simulink model "nonlineardtm"  (R2018b)
settings: configuration reference "Physics" (kept outside this file)
model workspace (MAT data in the model file):
  x0_initialstates = Simulink.Parameter
  x0_initialstates.Value = [0 0 0 0 0 0]
  x0_initialstates.DataType = 'auto'
  x0_initialstates.Dimensions = [1 6]
undefined symbols (not defined in the file): INIT__initialvalues__Vehicle_InitialPitchAngle, INIT__initialvalues__Vehicle_InitialPitchRate_radps, INIT__initialvalues__Vehicle_InitialVelocity_mps__2, INIT__initialvalues__Vehicle_InitialVelocity_mps__3, INIT__initialvalues__Vehicle_InitialYawAngle, INIT__initialvalues__Vehicle_InitialYawRate_radps, tireFL__INERTIAL__m_Wheel_kg, tireFL__SCALING__LCX, tireFL__SCALING__LCY, tireFL__SCALING__LCZ, tireFL__SCALING__LEX, tireFL__SCALING__LEY, tireFL__SCALING__LFZO, tireFL__SCALING__LGAY, tireFL__SCALING__LGAZ, tireFL__SCALING__LHX, tireFL__SCALING__LHY, tireFL__SCALING__LKX, tireFL__SCALING__LKY, tireFL__SCALING__LMPHI, tireFL__SCALING__LMUV, tireFL__SCALING__LMX, tireFL__SCALING__LMY, tireFL__SCALING__LRES, tireFL__SCALING__LS, tireFL__SCALING__LTR, tireFL__SCALING__LVMX, tireFL__SCALING__LVX, tireFL__SCALING__LVY, tireFL__SCALING__LVYKA, tireFL__SCALING__LXAL, tireFL__SCALING__LYKA, tireFR__INERTIAL__m_Wheel_kg, tireFR__SCALING__LCX, tireFR__SCALING__LCY, tireFR__SCALING__LCZ, tireFR__SCALING__LEX, tireFR__SCALING__LEY, tireFR__SCALING__LFZO, tireFR__SCALING__LGAY, tireFR__SCALING__LGAZ, tireFR__SCALING__LHX, tireFR__SCALING__LHY, tireFR__SCALING__LKX, tireFR__SCALING__LKY, tireFR__SCALING__LMPHI, tireFR__SCALING__LMUV, tireFR__SCALING__LMX, tireFR__SCALING__LMY, tireFR__SCALING__LRES, tireFR__SCALING__LS, tireFR__SCALING__LTR, tireFR__SCALING__LVMX, tireFR__SCALING__LVX, tireFR__SCALING__LVY, tireFR__SCALING__LVYKA, tireFR__SCALING__LXAL, tireFR__SCALING__LYKA, tireRL__INERTIAL__m_Wheel_kg, tireRL__SCALING__LCX ... (+71)
libraries: vehdynlibtire_TUM x4, vehdynlibsuspension x2, vrlib x1, vehdynlibeom_TUM x1
(part 1 of 5)
settings Model: DataDictionary=vehicleparameters_vehdynsim.sldd  ParameterArgumentNames=x0_initialstates  OrderedModelArguments=off  Creator=wischnewski  LastModifiedBy=Michael

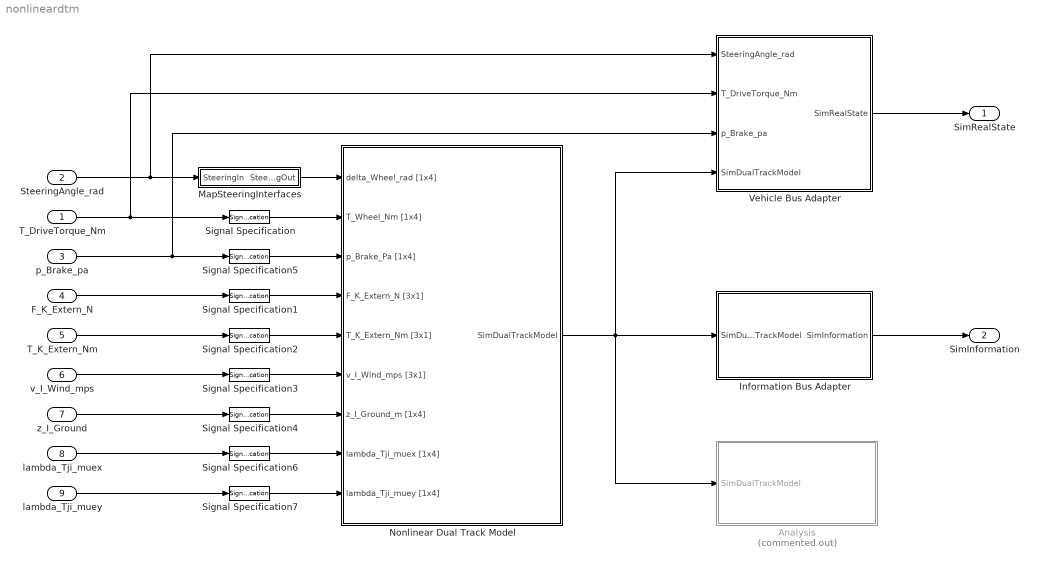
== system nonlineardtm ==
  T_DriveTorque_Nm : Inport  OutDataTypeStr=double
  SteeringAngle_rad : Inport  Port=2  OutDataTypeStr=double
  p_Brake_pa : Inport  Port=3  OutDataTypeStr=double
  F_K_Extern_N : Inport  Port=4  OutDataTypeStr=double
  T_K_Extern_Nm : Inport  Port=5  OutDataTypeStr=double
  v_I_Wind_mps : Inport  Port=6  OutDataTypeStr=double
  z_I_Ground : Inport  Port=7  OutDataTypeStr=double
  lambda_Tji_muex : Inport  Port=8  OutDataTypeStr=double
  lambda_Tji_muey : Inport  Port=9  OutDataTypeStr=double
  Analysis : Subsystem  Commented=on
  Information Bus Adapter : Subsystem
  MapSteeringInterfaces : Subsystem
  Nonlinear Dual Track Model : Subsystem
  Signal Specification{,4..7} (5 alike) : SignalSpecification  Dimensions=[1,4]
  Signal Specification1 : SignalSpecification  Dimensions=[3,1]
  Signal Specification2 : SignalSpecification  Dimensions=[3,1]
  Signal Specification3 : SignalSpecification  Dimensions=[3,1]
  Vehicle Bus Adapter : Subsystem
  SimRealState : Outport  OutDataTypeStr=Bus: SimRealState
  SimInformation : Outport  Port=2  OutDataTypeStr=Bus: SimInformation
  wires:
  Vehicle Bus Adapter/1(SimRealState) -> SimRealState/1
  Nonlinear Dual Track Model/1(SimDualTrackModel) -> Vehicle Bus Adapter/4(SimDualTrackModel), Information Bus Adapter/1(SimDualTrackModel), Analysis/1(SimDualTrackModel)
  Information Bus Adapter/1(SimInformation) -> SimInformation/1
  F_K_Extern_N/1 -> Signal Specification1/1
  T_K_Extern_Nm/1 -> Signal Specification2/1
  v_I_Wind_mps/1 -> Signal Specification3/1
  z_I_Ground/1 -> Signal Specification4/1
  lambda_Tji_muex/1 -> Signal Specification6/1
  lambda_Tji_muey/1 -> Signal Specification7/1
  p_Brake_pa/1 -> Signal Specification5/1, Vehicle Bus Adapter/3("p_Brake_pa ")
  T_DriveTorque_Nm/1 -> Vehicle Bus Adapter/2(T_DriveTorque_Nm), Signal Specification/1
  MapSteeringInterfaces/1(SteeringOut) -> Nonlinear Dual Track Model/1(delta_Wheel_rad [1x4])
  SteeringAngle_rad/1 -> Vehicle Bus Adapter/1(SteeringAngle_rad), MapSteeringInterfaces/1(SteeringIn)
  Signal Specification/1 -> Nonlinear Dual Track Model/2(T_Wheel_Nm [1x4])
  Signal Specification1/1 -> Nonlinear Dual Track Model/4(F_K_Extern_N [3x1])
  Signal Specification2/1 -> Nonlinear Dual Track Model/5(T_K_Extern_Nm [3x1])
  Signal Specification3/1 -> Nonlinear Dual Track Model/6(v_I_Wind_mps [3x1])
  Signal Specification4/1 -> Nonlinear Dual Track Model/7(z_I_Ground_m [1x4])
  Signal Specification5/1 -> Nonlinear Dual Track Model/3(p_Brake_Pa [1x4])
  Signal Specification6/1 -> Nonlinear Dual Track Model/8(lambda_Tji_muex [1x4])
  Signal Specification7/1 -> Nonlinear Dual Track Model/9(lambda_Tji_muey [1x4])

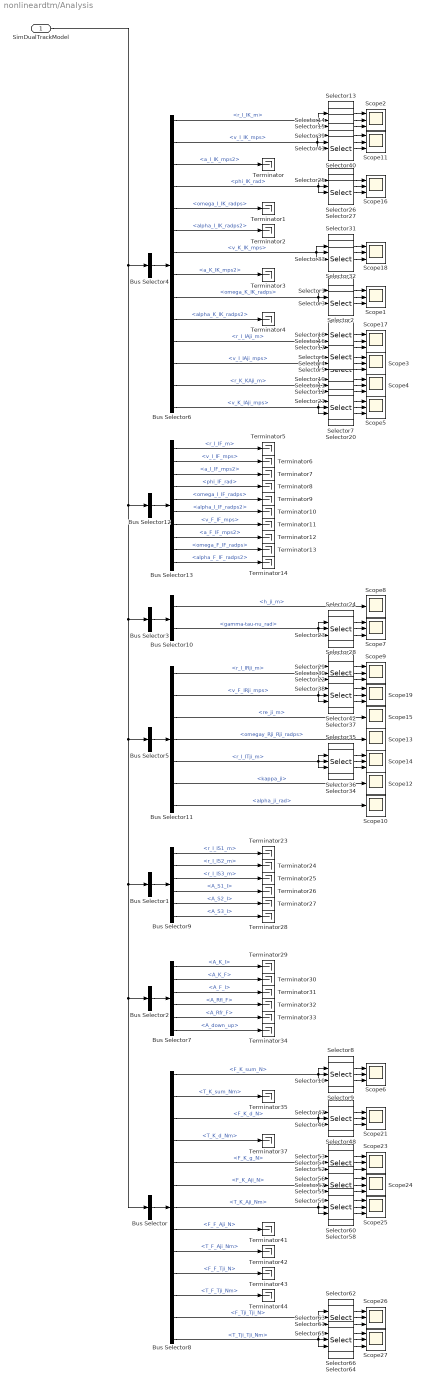
== system nonlineardtm/Analysis ==
  SimDualTrackModel : Inport
  Bus Selector : BusSelector  OutputSignals=SimForce  OutputAsBus=on
  Bus Selector1 : BusSelector  OutputSignals=SimSensor  OutputAsBus=on
  Bus Selector10 : BusSelector  OutputSignals=h_ji_m,gamma-tau-nu_rad
  Bus Selector11 : BusSelector  OutputSignals=r_I_IRji_m,v_F_IRji_mps,re_ji_m,omegay_Rji_Rji_radps,r_I_ITji_m,kappa_ji,alpha_ji_rad
  Bus Selector12 : BusSelector  OutputSignals=SimChassis  OutputAsBus=on
  Bus Selector13 : BusSelector  OutputSignals=r_I_IF_m,v_I_IF_mps,a_I_IF_mps2,phi_IF_rad,omega_I_IF_radps,alpha_I_IF_radps2,v_F_IF_mps,a_F_IF_mps2,omega_F_IF_radps,alpha_F_IF_radps2
  Bus Selector2 : BusSelector  OutputSignals=signal6  OutputAsBus=on
  Bus Selector3 : BusSelector  OutputSignals=SimSuspension  OutputAsBus=on
  Bus Selector4 : BusSelector  OutputSignals=signal1  OutputAsBus=on
  Bus Selector5 : BusSelector  OutputSignals=SimWheel  OutputAsBus=on
  Bus Selector6 : BusSelector  OutputSignals=r_I_IK_m,v_I_IK_mps,a_I_IK_mps2,phi_IK_rad,omega_I_IK_radps,alpha_I_IK_radps2,v_K_IK_mps,a_K_IK_mps2,omega_K_IK_radps,alpha_K_IK_radps2,r_I_IAji_m,v_I_IAji_mps,r_K_KAji_m,v_K_IAji_mps
  Bus Selector7 : BusSelector  OutputSignals=A_K_I,A_K_F,A_F_I,A_Rfl_F,A_Rfr_F,A_down_up
  Bus Selector8 : BusSelector  OutputSignals=F_K_sum_N,T_K_sum_Nm,F_K_d_N,T_K_d_Nm,F_K_g_N,F_K_Aji_N,T_K_Aji_Nm,F_F_Aji_N,T_F_Aji_Nm,F_F_Tji_N,T_F_Tji_Nm,F_Tji_Tji_N,T_Tji_Tji_Nm
  Bus Selector9 : BusSelector  OutputSignals=r_I_IS1_m,r_I_IS2_m,r_I_IS3_m,A_S1_I,A_S2_I,A_S3_I
  Scope{1..7,9,11,14,16..19,21,23..27} (20 alike) : Scope  NumInputPorts=3
  Scope{8,10,12..13,15} (5 alike) : Scope
  Selector{1,8,13,25,31,39,47,53} (8 alike) : Selector  InputPortWidth=3  IndexOptions=Index vector (dialog)  Indices=[1]  OutputSizes=1
  Selector{3,10,15,27,33,41,46,52} (8 alike) : Selector  InputPortWidth=3  IndexOptions=Index vector (dialog)  Indices=[3]  OutputSizes=1
  Selector{4,7,11,16,28,30,36,42,57,60,63,66} (12 alike) : Selector  NumberOfDimensions=2  InputPortWidth=3  IndexOptions=Index vector (dialog),Select all  Indices=2,1  OutputSizes=1,1
  Selector{5,12,17,20,22..23,34,37,55,58,61,64} (12 alike) : Selector  NumberOfDimensions=2  InputPortWidth=3  IndexOptions=Index vector (dialog),Select all  Indices=3,1  OutputSizes=1,1
  Selector{2,9,14,26,32,40,48,54} (8 alike) : Selector  InputPortWidth=3  IndexOptions=Index vector (dialog)  Indices=[2]  OutputSizes=1
  Selector{6,18..19,21,24,29,35,38,56,59,62,65} (12 alike) : Selector  NumberOfDimensions=2  InputPortWidth=3  IndexOptions=Index vector (dialog),Select all  Indices=1,1  OutputSizes=1,1
  Terminator{,1..14,23..35,37,41..44} (33 alike) : Terminator
  wires:
  SimDualTrackModel/1 -> Bus Selector12/1, Bus Selector5/1, Bus Selector/1, Bus Selector2/1, Bus Selector1/1, Bus Selector3/1, Bus Selector4/1
  Bus Selector12/1 -> Bus Selector13/1
  Bus Selector13/1 -> Terminator5/1  "<r_I_IF_m>"
  Bus Selector13/2 -> Terminator6/1  "<v_I_IF_mps>"
  Bus Selector13/3 -> Terminator7/1  "<a_I_IF_mps2>"
  Bus Selector13/4 -> Terminator8/1  "<phi_IF_rad>"
  Bus Selector13/5 -> Terminator9/1  "<omega_I_IF_radps>"
  Bus Selector13/6 -> Terminator10/1  "<alpha_I_IF_radps2>"
  Bus Selector13/7 -> Terminator11/1  "<v_F_IF_mps>"
  Bus Selector13/8 -> Terminator12/1  "<a_F_IF_mps2>"
  Bus Selector13/9 -> Terminator13/1  "<omega_F_IF_radps>"
  Bus Selector13/10 -> Terminator14/1  "<alpha_F_IF_radps2>"
  Bus Selector11/6 -> Scope12/1  "<kappa_ji>"
  Bus Selector11/7 -> Scope10/1  "<alpha_ji_rad>"
  Bus Selector11/4 -> Scope13/1  "<omegay_Rji_Rji_radps>"
  Bus Selector11/3 -> Scope15/1  "<re_ji_m>"
  Bus Selector11/1 -> Selector29/1, Selector30/1, Selector22/1  "<r_I_IRji_m>"
  Bus Selector5/1 -> Bus Selector11/1
  Bus Selector10/1 -> Scope8/1  "<h_ji_m>"
  Bus Selector3/1 -> Bus Selector10/1
  Bus Selector6/11 -> Selector16/1, Selector17/1, Selector18/1  "<r_I_IAji_m>"
  Bus Selector6/10 -> Terminator4/1  "<alpha_K_IK_radps2>"
  Bus Selector6/9 -> Selector2/1, Selector3/1, Selector1/1  "<omega_K_IK_radps>"
  Bus Selector6/8 -> Terminator3/1  "<a_K_IK_mps2>"
  Bus Selector6/7 -> Selector33/1, Selector32/1, Selector31/1  "<v_K_IK_mps>"
  Bus Selector6/6 -> Terminator2/1  "<alpha_I_IK_radps2>"
  Bus Selector6/5 -> Terminator1/1  "<omega_I_IK_radps>"
  Bus Selector6/4 -> Selector25/1, Selector27/1, Selector26/1  "<phi_IK_rad>"
  Bus Selector6/3 -> Terminator/1  "<a_I_IK_mps2>"
  Bus Selector6/2 -> Selector39/1, Selector41/1, Selector40/1  "<v_I_IK_mps>"
  Bus Selector6/1 -> Selector13/1, Selector15/1, Selector14/1  "<r_I_IK_m>"
  Bus Selector9/5 -> Terminator27/1  "<A_S2_I>"
  Bus Selector9/4 -> Terminator26/1  "<A_S1_I>"
  Bus Selector9/3 -> Terminator25/1  "<r_I_IS3_m>"
  Bus Selector9/2 -> Terminator24/1  "<r_I_IS2_m>"
  Bus Selector9/1 -> Terminator23/1  "<r_I_IS1_m>"
  Bus Selector9/6 -> Terminator28/1  "<A_S3_I>"
  Bus Selector1/1 -> Bus Selector9/1
  Bus Selector8/11 -> Terminator44/1  "<T_F_Tji_Nm>"
  Bus Selector8/10 -> Terminator43/1  "<F_F_Tji_N>"
  Bus Selector8/9 -> Terminator42/1  "<T_F_Aji_Nm>"
  Bus Selector8/8 -> Terminator41/1  "<F_F_Aji_N>"
  Bus Selector8/6 -> Selector57/1, Selector56/1, Selector55/1  "<F_K_Aji_N>"
  Bus Selector8/4 -> Terminator37/1  "<T_K_d_Nm>"
  Bus Selector8/2 -> Terminator35/1  "<T_K_sum_Nm>"
  Bus Selector/1 -> Bus Selector8/1
  Bus Selector7/6 -> Terminator34/1  "<A_down_up>"
  Bus Selector7/5 -> Terminator33/1  "<A_Rfr_F>"
  Bus Selector7/4 -> Terminator32/1  "<A_Rfl_F>"
  Bus Selector7/3 -> Terminator31/1  "<A_F_I>"
  Bus Selector7/2 -> Terminator30/1  "<A_K_F>"
  Bus Selector7/1 -> Terminator29/1  "<A_K_I>"
  Bus Selector2/1 -> Bus Selector7/1
  Bus Selector4/1 -> Bus Selector6/1
  Selector32/1 -> Scope18/2
  Selector40/1 -> Scope11/2
  Selector31/1 -> Scope18/1
  Selector13/1 -> Scope2/1
  Selector15/1 -> Scope2/3
  Selector26/1 -> Scope16/2
  Selector16/1 -> Scope17/2
  Selector27/1 -> Scope16/3
  Selector17/1 -> Scope17/3
  Selector33/1 -> Scope18/3
  Selector25/1 -> Scope16/1
  Selector18/1 -> Scope17/1
  Selector41/1 -> Scope11/3
  Selector39/1 -> Scope11/1
  Selector14/1 -> Scope2/2
  Selector1/1 -> Scope1/1
  Selector3/1 -> Scope1/3
  Selector2/1 -> Scope1/2
  Selector6/1 -> Scope3/1
  Selector5/1 -> Scope3/3
  Selector4/1 -> Scope3/2
  Bus Selector6/12 -> Selector6/1, Selector5/1, Selector4/1  "<v_I_IAji_mps>"
  Bus Selector6/13 -> Selector19/1, Selector11/1, Selector12/1  "<r_K_KAji_m>"
  Selector11/1 -> Scope4/2
  Selector12/1 -> Scope4/3
  Selector19/1 -> Scope4/1
  Selector21/1 -> Scope5/1
  Selector20/1 -> Scope5/3
  Selector7/1 -> Scope5/2
  Bus Selector6/14 -> Selector20/1, Selector7/1, Selector21/1  "<v_K_IAji_mps>"
  Selector9/1 -> Scope6/2
  Selector10/1 -> Scope6/3
  Selector8/1 -> Scope6/1
  Bus Selector8/1 -> Selector8/1, Selector9/1, Selector10/1  "<F_K_sum_N>"
  Bus Selector10/2 -> Selector23/1, Selector24/1, Selector28/1  "<gamma-tau-nu_rad>"
  Selector28/1 -> Scope7/2
  Selector23/1 -> Scope7/3
  Selector24/1 -> Scope7/1
  Selector29/1 -> Scope9/1
  Selector22/1 -> Scope9/3
  Selector30/1 -> Scope9/2
  Bus Selector11/5 -> Selector34/1, Selector35/1, Selector36/1  "<r_I_ITji_m>"
  Selector36/1 -> Scope14/2
  Selector34/1 -> Scope14/3
  Selector35/1 -> Scope14/1
  Bus Selector11/2 -> Selector37/1, Selector38/1, Selector42/1  "<v_F_IRji_mps>"
  Selector42/1 -> Scope19/2
  Selector37/1 -> Scope19/3
  Selector38/1 -> Scope19/1
  Bus Selector8/3 -> Selector47/1, Selector46/1, Selector48/1  "<F_K_d_N>"
  Selector47/1 -> Scope21/1
  Selector46/1 -> Scope21/3
  Selector48/1 -> Scope21/2
  Selector54/1 -> Scope23/2
  Selector52/1 -> Scope23/3
  Selector53/1 -> Scope23/1
  Bus Selector8/5 -> Selector54/1, Selector52/1, Selector53/1  "<F_K_g_N>"
  Selector56/1 -> Scope24/1
  Selector55/1 -> Scope24/3
  Selector57/1 -> Scope24/2
  Selector60/1 -> Scope25/2
  Selector58/1 -> Scope25/3
  Selector59/1 -> Scope25/1
  Bus Selector8/7 -> Selector58/1, Selector59/1, Selector60/1  "<T_K_Aji_Nm>"
  Bus Selector8/12 -> Selector63/1, Selector62/1, Selector61/1  "<F_Tji_Tji_N>"
  Selector62/1 -> Scope26/1
  Selector61/1 -> Scope26/3
  Selector63/1 -> Scope26/2
  Selector66/1 -> Scope27/2
  Selector64/1 -> Scope27/3
  Selector65/1 -> Scope27/1
  Bus Selector8/13 -> Selector64/1, Selector65/1, Selector66/1  "<T_Tji_Tji_Nm>"

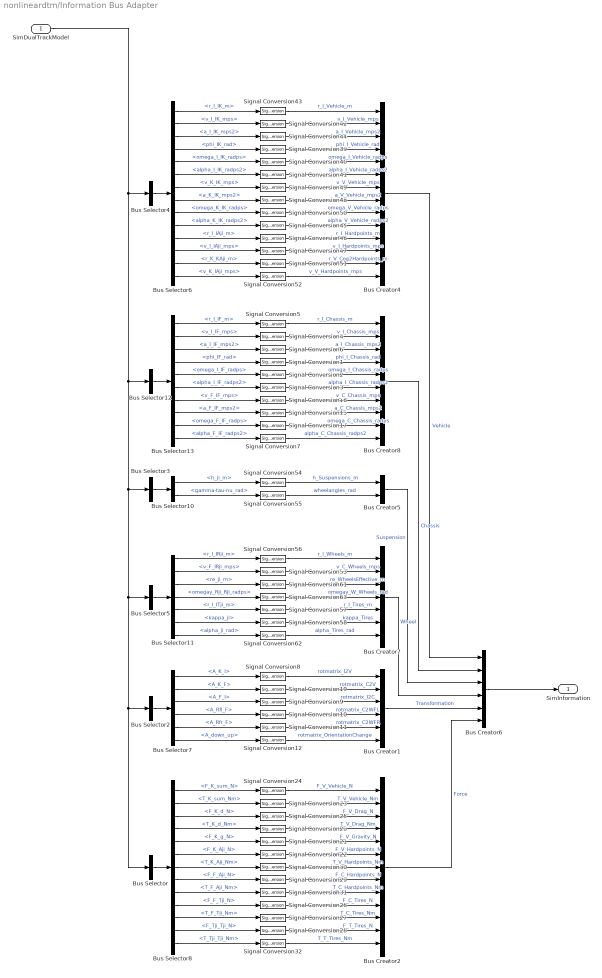
== system nonlineardtm/Information Bus Adapter ==
  SimDualTrackModel : Inport
  Bus Creator1 : BusCreator  Inputs=6  OutDataTypeStr=Bus: Transformation
      settings: InheritFromInputs=off
  Bus Creator2 : BusCreator  Inputs=13  OutDataTypeStr=Bus: Force
      settings: InheritFromInputs=off
  Bus Creator4 : BusCreator  Inputs=14  OutDataTypeStr=Bus: Vehicle
      settings: InheritFromInputs=off
  Bus Creator5 : BusCreator  Inputs=2  OutDataTypeStr=Bus: Suspension
      settings: InheritFromInputs=off
  Bus Creator6 : BusCreator  Inputs=6  OutDataTypeStr=Bus: SimInformation
      settings: InheritFromInputs=off
  Bus Creator7 : BusCreator  Inputs=7  OutDataTypeStr=Bus: Wheel
      settings: InheritFromInputs=off
  Bus Creator8 : BusCreator  Inputs=10  OutDataTypeStr=Bus: Chassis
      settings: InheritFromInputs=off
  Bus Selector : BusSelector  OutputSignals=SimForce  OutputAsBus=on
  Bus Selector10 : BusSelector  OutputSignals=h_ji_m,gamma-tau-nu_rad
  Bus Selector11 : BusSelector  OutputSignals=r_I_IRji_m,v_F_IRji_mps,re_ji_m,omegay_Rji_Rji_radps,r_I_ITji_m,kappa_ji,alpha_ji_rad
  Bus Selector12 : BusSelector  OutputSignals=SimChassis  OutputAsBus=on
  Bus Selector13 : BusSelector  OutputSignals=r_I_IF_m,v_I_IF_mps,a_I_IF_mps2,phi_IF_rad,omega_I_IF_radps,alpha_I_IF_radps2,v_F_IF_mps,a_F_IF_mps2,omega_F_IF_radps,alpha_F_IF_radps2
  Bus Selector2 : BusSelector  OutputSignals=signal5  OutputAsBus=on
  Bus Selector3 : BusSelector  OutputSignals=SimSuspension  OutputAsBus=on
  Bus Selector4 : BusSelector  OutputSignals=signal1  OutputAsBus=on
  Bus Selector5 : BusSelector  OutputSignals=SimWheel  OutputAsBus=on
  Bus Selector6 : BusSelector  OutputSignals=r_I_IK_m,v_I_IK_mps,a_I_IK_mps2,phi_IK_rad,omega_I_IK_radps,alpha_I_IK_radps2,v_K_IK_mps,a_K_IK_mps2,omega_K_IK_radps,alpha_K_IK_radps2,r_I_IAji_m,v_I_IAji_mps,r_K_KAji_m,v_K_IAji_mps
  Bus Selector7 : BusSelector  OutputSignals=A_K_I,A_K_F,A_F_I,A_Rfl_F,A_Rfr_F,A_down_up
  Bus Selector8 : BusSelector  OutputSignals=F_K_sum_N,T_K_sum_Nm,F_K_d_N,T_K_d_Nm,F_K_g_N,F_K_Aji_N,T_K_Aji_Nm,F_F_Aji_N,T_F_Aji_Nm,F_F_Tji_N,T_F_Tji_Nm,F_Tji_Tji_N,T_Tji_Tji_Nm
  Signal Conversion{1..12,15..17,19..32,39..58,61..63} (52 alike) : SignalConversion  OverrideOpt=off
  SimInformation : Outport  OutDataTypeStr=Bus: SimInformation
  wires:
  Bus Selector4/1 -> Bus Selector6/1
  Bus Selector2/1 -> Bus Selector7/1
  Bus Selector7/1 -> Signal Conversion8/1  "<A_K_I>"
  Bus Selector7/2 -> Signal Conversion19/1  "<A_K_F>"
  Bus Selector7/3 -> Signal Conversion9/1  "<A_F_I>"
  Bus Selector7/4 -> Signal Conversion10/1  "<A_Rfl_F>"
  Bus Selector7/5 -> Signal Conversion11/1  "<A_Rfr_F>"
  Bus Selector7/6 -> Signal Conversion12/1  "<A_down_up>"
  Signal Conversion8/1 -> Bus Creator1/1  "rotmatrix_I2V"
  Signal Conversion19/1 -> Bus Creator1/2  "rotmatrix_C2V"
  Signal Conversion9/1 -> Bus Creator1/3  "rotmatrix_I2C"
  Signal Conversion10/1 -> Bus Creator1/4  "rotmatrix_C2WFL"
  Signal Conversion11/1 -> Bus Creator1/5  "rotmatrix_C2WFR"
  Signal Conversion12/1 -> Bus Creator1/6  "rotmatrix_OrientationChange"
  Bus Selector/1 -> Bus Selector8/1
  Bus Selector8/1 -> Signal Conversion24/1  "<F_K_sum_N>"
  Bus Selector8/2 -> Signal Conversion23/1  "<T_K_sum_Nm>"
  Bus Selector8/3 -> Signal Conversion25/1  "<F_K_d_N>"
  Bus Selector8/4 -> Signal Conversion20/1  "<T_K_d_Nm>"
  Bus Selector8/5 -> Signal Conversion21/1  "<F_K_g_N>"
  Bus Selector8/6 -> Signal Conversion22/1  "<F_K_Aji_N>"
  Bus Selector8/7 -> Signal Conversion30/1  "<T_K_Aji_Nm>"
  Bus Selector8/8 -> Signal Conversion29/1  "<F_F_Aji_N>"
  Bus Selector8/9 -> Signal Conversion31/1  "<T_F_Aji_Nm>"
  Bus Selector8/10 -> Signal Conversion26/1  "<F_F_Tji_N>"
  Bus Selector8/11 -> Signal Conversion27/1  "<T_F_Tji_Nm>"
  Bus Selector8/12 -> Signal Conversion28/1  "<F_Tji_Tji_N>"
  Bus Selector8/13 -> Signal Conversion32/1  "<T_Tji_Tji_Nm>"
  Signal Conversion23/1 -> Bus Creator2/2  "T_V_Vehicle_Nm"
  Signal Conversion24/1 -> Bus Creator2/1  "F_V_Vehicle_N"
  Signal Conversion25/1 -> Bus Creator2/3  "F_V_Drag_N"
  Signal Conversion20/1 -> Bus Creator2/4  "T_V_Drag_Nm"
  Signal Conversion21/1 -> Bus Creator2/5  "F_V_Gravity_N"
  Signal Conversion22/1 -> Bus Creator2/6  "F_V_Hardpoints_N"
  Signal Conversion30/1 -> Bus Creator2/7  "T_V_Hardpoints_Nm"
  Signal Conversion29/1 -> Bus Creator2/8  "F_C_Hardpoints_N"
  Signal Conversion31/1 -> Bus Creator2/9  "T_C_Hardpoints_Nm"
  Signal Conversion26/1 -> Bus Creator2/10  "F_C_Tires_N"
  Signal Conversion27/1 -> Bus Creator2/11  "T_C_Tires_Nm"
  Signal Conversion28/1 -> Bus Creator2/12  "F_T_Tires_N"
  Signal Conversion32/1 -> Bus Creator2/13  "T_T_Tires_Nm"
  Bus Selector6/1 -> Signal Conversion43/1  "<r_I_IK_m>"
  Bus Selector6/2 -> Signal Conversion42/1  "<v_I_IK_mps>"
  Bus Selector6/3 -> Signal Conversion44/1  "<a_I_IK_mps2>"
  Bus Selector6/4 -> Signal Conversion39/1  "<phi_IK_rad>"
  Bus Selector6/5 -> Signal Conversion40/1  "<omega_I_IK_radps>"
  Bus Selector6/6 -> Signal Conversion41/1  "<alpha_I_IK_radps2>"
  Bus Selector6/7 -> Signal Conversion49/1  "<v_K_IK_mps>"
  Bus Selector6/8 -> Signal Conversion48/1  "<a_K_IK_mps2>"
  Bus Selector6/9 -> Signal Conversion50/1  "<omega_K_IK_radps>"
  Bus Selector6/10 -> Signal Conversion45/1  "<alpha_K_IK_radps2>"
  Bus Selector6/11 -> Signal Conversion46/1  "<r_I_IAji_m>"
  Bus Selector6/12 -> Signal Conversion47/1  "<v_I_IAji_mps>"
  Bus Selector6/14 -> Signal Conversion52/1  "<v_K_IAji_mps>"
  Bus Selector6/13 -> Signal Conversion51/1  "<r_K_KAji_m>"
  Signal Conversion43/1 -> Bus Creator4/1  "r_I_Vehicle_m"
  Signal Conversion42/1 -> Bus Creator4/2  "v_I_Vehicle_mps"
  Signal Conversion44/1 -> Bus Creator4/3  "a_I_Vehicle_mps2"
  Signal Conversion39/1 -> Bus Creator4/4  "phi_I_Vehicle_rad"
  Signal Conversion40/1 -> Bus Creator4/5  "omega_I_Vehicle_radps"
  Signal Conversion41/1 -> Bus Creator4/6  "alpha_I_Vehicle_radps2"
  Signal Conversion49/1 -> Bus Creator4/7  "v_V_Vehicle_mps"
  Signal Conversion48/1 -> Bus Creator4/8  "a_V_Vehicle_mps2"
  Signal Conversion50/1 -> Bus Creator4/9  "omega_V_Vehicle_radps"
  Signal Conversion45/1 -> Bus Creator4/10  "alpha_V_Vehicle_radps2"
  Signal Conversion46/1 -> Bus Creator4/11  "r_I_Hardpoints_m"
  Signal Conversion47/1 -> Bus Creator4/12  "v_I_Hardpoints_mps"
  Signal Conversion51/1 -> Bus Creator4/13  "r_V_Cog2Hardpoints_m"
  Signal Conversion52/1 -> Bus Creator4/14  "v_V_Hardpoints_mps"
  Bus Selector3/1 -> Bus Selector10/1
  Signal Conversion55/1 -> Bus Creator5/2  "wheelangles_rad"
  Signal Conversion54/1 -> Bus Creator5/1  "h_Suspensions_m"
  Signal Conversion53/1 -> Bus Creator7/2  "v_C_Wheels_mps"
  Bus Selector10/1 -> Signal Conversion54/1  "<h_ji_m>"
  Bus Selector10/2 -> Signal Conversion55/1  "<gamma-tau-nu_rad>"
  Bus Selector11/2 -> Signal Conversion53/1  "<v_F_IRji_mps>"
  Bus Selector5/1 -> Bus Selector11/1
  Signal Conversion63/1 -> Bus Creator7/4  "omegay_W_Wheels_rad"
  Signal Conversion62/1 -> Bus Creator7/7  "alpha_Tires_rad"
  Signal Conversion58/1 -> Bus Creator7/6  "kappa_Tires"
  Signal Conversion57/1 -> Bus Creator7/5  "r_I_Tires_m"
  Signal Conversion56/1 -> Bus Creator7/1  "r_I_Wheels_m"
  Signal Conversion61/1 -> Bus Creator7/3  "re_WheelsEffective_m"
  Bus Selector11/1 -> Signal Conversion56/1  "<r_I_IRji_m>"
  Bus Selector11/3 -> Signal Conversion61/1  "<re_ji_m>"
  Bus Selector11/4 -> Signal Conversion63/1  "<omegay_Rji_Rji_radps>"
  Bus Selector11/7 -> Signal Conversion62/1  "<alpha_ji_rad>"
  Bus Selector11/6 -> Signal Conversion58/1  "<kappa_ji>"
  Bus Selector11/5 -> Signal Conversion57/1  "<r_I_ITji_m>"
  Bus Creator4/1 -> Bus Creator6/1  "Vehicle"
  Bus Creator7/1 -> Bus Creator6/4  "Wheel"
  Bus Creator1/1 -> Bus Creator6/5  "Transformation"
  Signal Conversion7/1 -> Bus Creator8/10  "alpha_C_Chassis_radps2"
  Signal Conversion17/1 -> Bus Creator8/9  "omega_C_Chassis_radps"
  Signal Conversion15/1 -> Bus Creator8/8  "a_C_Chassis_mps2"
  Signal Conversion16/1 -> Bus Creator8/7  "v_C_Chassis_mps"
  Signal Conversion3/1 -> Bus Creator8/6  "alpha_I_Chassis_radps2"
  Signal Conversion2/1 -> Bus Creator8/5  "omega_I_Chassis_radps"
  Signal Conversion1/1 -> Bus Creator8/4  "phi_I_Chassis_rad"
  Signal Conversion6/1 -> Bus Creator8/3  "a_I_Chassis_mps2"
  Signal Conversion4/1 -> Bus Creator8/2  "v_I_Chassis_mps"
  Signal Conversion5/1 -> Bus Creator8/1  "r_I_Chassis_m"
  Bus Selector13/10 -> Signal Conversion7/1  "<alpha_F_IF_radps2>"
  Bus Selector13/9 -> Signal Conversion17/1  "<omega_F_IF_radps>"
  Bus Selector13/8 -> Signal Conversion15/1  "<a_F_IF_mps2>"
  Bus Selector13/7 -> Signal Conversion16/1  "<v_F_IF_mps>"
  Bus Selector13/6 -> Signal Conversion3/1  "<alpha_I_IF_radps2>"
  Bus Selector13/5 -> Signal Conversion2/1  "<omega_I_IF_radps>"
  Bus Selector13/4 -> Signal Conversion1/1  "<phi_IF_rad>"
  Bus Selector13/3 -> Signal Conversion6/1  "<a_I_IF_mps2>"
  Bus Selector13/2 -> Signal Conversion4/1  "<v_I_IF_mps>"
  Bus Selector13/1 -> Signal Conversion5/1  "<r_I_IF_m>"
  Bus Selector12/1 -> Bus Selector13/1
  SimDualTrackModel/1 -> Bus Selector4/1, Bus Selector/1, Bus Selector2/1, Bus Selector5/1, Bus Selector3/1, Bus Selector12/1
  Bus Creator8/1 -> Bus Creator6/2  "Chassis"
  Bus Creator2/1 -> Bus Creator6/6  "Force"
  Bus Creator5/1 -> Bus Creator6/3  "Suspension"
  Bus Creator6/1 -> SimInformation/1

== system nonlineardtm/MapSteeringInterfaces ==
  SteeringIn : Inport  PortDimensions=1
  Constant : Constant  Value=0
  Gain : Gain  Gain=-1
  Mux : Mux
  SteeringOut : Outport
  wires:
  SteeringIn/1 -> Gain/1
  Mux/1 -> SteeringOut/1
  Constant/1 -> Mux/3, Mux/4
  Gain/1 -> Mux/2, Mux/1

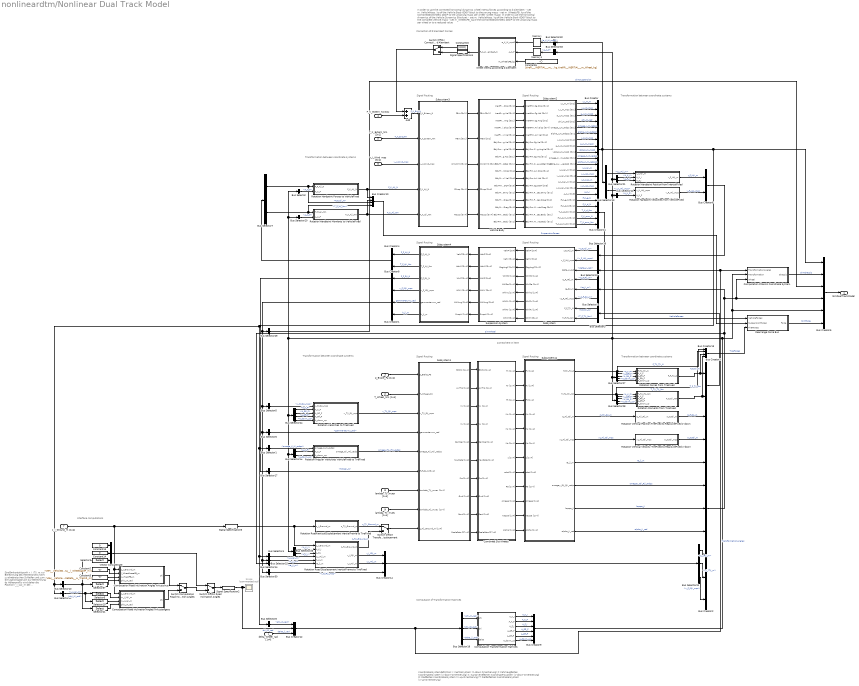
== system nonlineardtm/Nonlinear Dual Track Model ==
  note: somewhere in here
  note: Straßenkontaktpunkt  r_I_ITji_m zur Berechnung des Höhhenprofils führt zu algebraischen Schleifen und zum Simulationsabbruch
      | Zur Berechnung ds Höhenprofils wird daher die Position r_I_IAji_m der Anbindungspunkte an die Radaufhängungen verwendet
      | Alternative: Einführung von Verzögerungsgliedern oder Memory-Blöcken
  note: Koordinatensystemdefinition:
      | I: Inertialsystem (z-down Orientierung)
      | F: Fahrzeugfestes Koordinatensystem (z-down-Orientierung)
      | K: Karosseriefestes Koordinatensystem (z-down-Orientierung)
      | R: Radfestes Koordinatensystem (z-up-Orientierung)
      | T: Reifenfestes Koordinatensystem (z-up-Orientierung)
  note: Transformation
      | between coordinate systems
  note: Signal Routing
  note: Signal Routing
  note: Signal Routing
  note: Signal Routing
  note: Transformation
      | between coordinate systems
  note: Signal Routing
  note: Signal Routing
  note: Transformation
      | between coordinate systems
  note: Transformation
      | between coordinate systems
  note: Interface computations
  note: Computaion of Transformation Matrices
  note: In order to use the corrected horizontal dynamics wheel inertia forces according to d'Alembert:
      | - set m_VehicleMass_kg of the Vehicle Body 6DOF block to the sprung mass
      | - set m_WheelsFB_kg of the CombinedSlipWheels 2DOF to the unsprung mass per wheel (wheel mass)
      | In order to use the horizontal dynamics of the Vehicle Dynamics Blockset:
      | - set m_VehicleMass_kg of the Vehicle Body 6DOF block to the complete vehicle mass
      | - set m_WheelsFB_kg of the CombinedSlipWheels 2DOF to the unsprung mass per wheel or to a reduced value
  note: Correction of d'Alembert Forces
  delta_Wheel_rad [1x4] : Inport
  T_Wheel_Nm [1x4] : Inport  Port=2
  p_Brake_Pa [1x4] : Inport  Port=3
  F_K_Extern_N [3x1] : Inport  Port=4
  T_K_Extern_Nm [3x1] : Inport  Port=5
  v_I_Wind_mps [3x1] : Inport  Port=6
  z_I_Ground_m [1x4] : Inport  Port=7
  lambda_Tji_muex [1x4] : Inport  Port=8
  lambda_Tji_muey [1x4] : Inport  Port=9
  Add : Sum
  Bus Creator : BusCreator  Inputs=16
  Bus Creator1 : BusCreator  Inputs=3
  Bus Creator10 : BusCreator  Inputs=4
  Bus Creator11 : BusCreator  Inputs=5
  Bus Creator12 : BusCreator  Inputs=3
  Bus Creator13 : BusCreator  Inputs=4
  Bus Creator14 : BusCreator  Inputs=3
  Bus Creator2 : BusCreator  Inputs=9
  Bus Creator3 : BusCreator  Inputs=2
  Bus Creator4 : BusCreator  Inputs=2
  Bus Creator5 : BusCreator  Inputs=6
  Bus Creator6 : BusCreator  Inputs=2
  Bus Creator8 : BusCreator  Inputs=1
  Bus Creator9 : BusCreator  Inputs=6
  Bus Selector{,12,20,33} (4 alike) : BusSelector  OutputSignals=A_K_F
  Bus Selector1 : BusSelector  OutputSignals=omega_K_IK_radps
  Bus Selector10 : BusSelector  OutputSignals=phi_IK_rad
  Bus Selector13 : BusSelector  OutputSignals=r_I_IAji_m,v_K_IAji_mps
  Bus Selector14 : BusSelector  OutputSignals=h_ji_m
  Bus Selector15 : BusSelector  OutputSignals=re_ji_m
  Bus Selector16 : BusSelector  OutputSignals=r_F_IAji_m,v_F_IAji_mps
  Bus Selector17 : BusSelector  OutputSignals=F_F_Rji_N
  Bus Selector19 : BusSelector  OutputSignals=phi_IK_rad,chi_IO_rad,delta_ji_rad
  Bus Selector2 : BusSelector  OutputSignals=rz_F_Rji_m,re_ji_m,vz_F_Rji_m
  Bus Selector21 : BusSelector  OutputSignals=A_K_I,A_F_I
  Bus Selector22 : BusSelector  OutputSignals=r_I_IAji_m
  Bus Selector23 : BusSelector  OutputSignals=delta_ji_rad
  Bus Selector24 : BusSelector  OutputSignals=A_K_F,A_Rfl_F,A_Rfr_F,A_down_up
  Bus Selector25 : BusSelector  OutputSignals=A_K_F,A_down_up
  Bus Selector26 : BusSelector  OutputSignals=A_K_I,A_F_I
  Bus Selector27 : BusSelector  OutputSignals=A_K_F,A_Rfl_F,A_Rfr_F,A_down_up
  Bus Selector28 : BusSelector  OutputSignals=A_K_F,A_Rfl_F,A_Rfr_F,A_down_up
  Bus Selector29 : BusSelector  OutputSignals=h_ji_m,gamma-tau-nu_rad  OutputAsBus=on
  Bus Selector3 : BusSelector  OutputSignals=F_F_Tji_N,T_F_Tji_Nm
  Bus Selector30 : BusSelector  OutputSignals=v_F_IRji_mps
  Bus Selector31 : BusSelector  OutputSignals=r_I_IRji_m,r_I_ITji_m,v_F_IRji_mps
  Bus Selector32 : BusSelector  OutputSignals=a_K_IK_mps2
  Bus Selector4 : BusSelector  OutputSignals=r_I_IAji_m
  Bus Selector5 : BusSelector  OutputSignals=v_F_IRji_mps
  Bus Selector6 : BusSelector  OutputSignals=gamma-tau-nu_rad
  Bus Selector7 : BusSelector  OutputSignals=F_F_Aji_N,T_F_Aji_Nm
  Bus Selector8 : BusSelector  OutputSignals=phi_IK_rad
  Combined Slip Wheels : Subsystem
  Computation Chassis Coordinate System : Subsystem
  Computation Road Inclination Angles Arkussinus : MATLAB Function  TreatAsAtomicUnit=on
  Computation Road Inclination Angles Arkustangens : MATLAB Function  TreatAsAtomicUnit=on
  Computation Transformation Matrices : MATLAB Function  TreatAsAtomicUnit=on
  Constant13 : Constant  Value=0
  Constant14 : Constant  Value=0
  Constant15 : Constant  Value=[0;0;0]
  Constant2 : Constant  Value="[VEH__VehicleData__l_WheelbaseF_m (VEH__VehicleData__l_WheelbaseTotal_m  - VEH__VehicleData__l_WheelbaseF_m)]"
  Constant5 : Constant  Value=[VEH__VehicleData__w_TrackF_m VEH__VehicleData__w_TrackR_m]
  Constant6 : Constant  Value=[tireFL__INERTIAL__m_Wheel_kg, tireFR__INERTIAL__m_Wheel_kg, tireRL__INERTIAL__m_Wheel_kg, tireRR__INERTIAL__m_Wheel_kg]
  Memory : Memory
  Memory1 : Memory
  Rearrange Force Bus : Subsystem
  Rotation Angular Velocities VehicleFixed to TireFixed : MATLAB Function  TreatAsAtomicUnit=on
  Rotation Forces from TireFixed : MATLAB Function  TreatAsAtomicUnit=on
  Rotation Hardpoint Forces to VehicleFixed : MATLAB Function  TreatAsAtomicUnit=on
  Rotation Hardpoint Moments to VehicleFixed : MATLAB Function  TreatAsAtomicUnit=on
  Rotation Hardpoint Position from InertialFixed : MATLAB Function  TreatAsAtomicUnit=on
  Rotation Hardpoint Velocities from VehicleFixed : MATLAB Function  TreatAsAtomicUnit=on
  Rotation Moments from TireFixed : MATLAB Function  TreatAsAtomicUnit=on
  Rotation Road Displacement InertialFrame to TireFixed : MATLAB Function  TreatAsAtomicUnit=on
  Rotation RoadVerticalDisplacement InertialFrame to TireFixed : Subsystem
  Rotation Velocities to TireFixed : MATLAB Function  TreatAsAtomicUnit=on
  Rotation Vertical Position TireFixed to RearAxleFixed z-down : Subsystem
  Rotation Vertical Velocity TireFixed to RearAxleFixed z-down : Subsystem
  Scope : Scope  Commented=on
  Selector20 : Selector  NumberOfDimensions=2  InputPortWidth=3  IndexOptions=Index vector (dialog),Select all  Indices=2,1  OutputSizes=1,1
  Selector21 : Selector  InputPortWidth=3  IndexOptions=Index vector (dialog)  Indices=3  OutputSizes=1
  Selector3 : Selector  InputPortWidth=3  IndexOptions=Index vector (dialog)  Indices=3  OutputSizes=1
  Selector37 : Selector  InputPortWidth=3  IndexOptions=Index vector (dialog)  Indices=3  OutputSizes=1
  Selector6 : Selector  NumberOfDimensions=2  InputPortWidth=3  IndexOptions=Index vector (dialog),Select all  Indices=1,1  OutputSizes=1,1
  Signal Specification2 : SignalSpecification  Dimensions=[3,1]
  Signal Specification4 : SignalSpecification  Dimensions=[3,1]
  Signal Specification5 : SignalSpecification  Dimensions=[1,4]
  Subsystem : Subsystem
  Subsystem1 : Subsystem
  Subsystem11 : Subsystem
  Subsystem2 : Subsystem
  Subsystem3 : Subsystem
  Subsystem4 : Subsystem
  Suspension System : Subsystem
  Switch Computation Road Inclination Angles : ManualSwitch
  Switch Off/On Correction Horizontal Dynamics Wheel Inertia according d'Alembert : ManualSwitch
  Switch Off/On Road Inclination Angles : ManualSwitch
  Switch Off/On Transformation Ground Displacement : ManualSwitch
  Vector Concatenate : Concatenate  NumInputs=3
  Vehicle Body : Subsystem
  Wheel Inertia according d'Alembert : MATLAB Function  TreatAsAtomicUnit=on
  SimDualTrackModel : Outport
  wires:
  Subsystem2/15(v_K_IAji_mps [3x4]) -> Bus Creator/15  "v_K_IAji_mps"
  Subsystem2/14(r_K_KAji_m [3x4]) -> Bus Creator/14  "r_K_KAji_m"
  Subsystem4/5(gamma-tau-nu_rad) -> Bus Creator1/2  "gamma-tau-nu_rad"
  Subsystem2/10(omega_K_IK_radps [3x1]) -> Bus Creator/10  "omega_K_IK_radps"
  Subsystem2/4(phi_IK_rad [3x1]) -> Bus Creator/4  "phi_IK_rad"
  v_I_Wind_mps [3x1]/1 -> Subsystem3/3(v_I_Wind_mps)  "v_I_Wind_mps"
  T_K_Extern_Nm [3x1]/1 -> Subsystem3/2(T_K_Extern_Nm)  "T_K_Ext_Nm"
  Add/1 -> Subsystem3/1(F_K_Extern_N)  "F_K_Ext_N"
  Subsystem11/6(omegay_Rji_Rji_radps) -> Bus Creator2/4  "omegay_Rji_Rji_radps"
  Subsystem11/4(vz_Tji_Rji_mps) -> Rotation Vertical Velocity TireFixed to RearAxleFixed z-down/1(vz_Tji_Rji_mps)  "vz_Tji_Rji_mps"
  Bus Creator2/1 -> Bus Selector2/1, Computation Chassis Coordinate System/3(Wheel), Bus Creator5/4, Bus Selector15/1  "SimWheel"
  Bus Selector2/1 -> Subsystem/4(rz_F_IRji_m)  "<rz_F_Rji_m>"
  Bus Selector2/2 -> Subsystem/5(re_Rji_m)  "<re_ji_m>"
  Bus Selector2/3 -> Subsystem/6(vz_F_IRji_mps)  "<vz_F_Rji_m>"
  Bus Creator3/1 -> Bus Selector3/1
  Bus Selector3/1 -> Subsystem/7(F_F_Tji_N)  "<F_F_Tji_N>"
  Bus Selector3/2 -> Subsystem/8(T_F_Tji_Nm)  "<T_F_Tji_Nm>"
  z_I_Ground_m [1x4]/1 -> Signal Specification5/1, Computation Road Inclination Angles Arkustangens/1(z_I_Ground_m), Computation Road Inclination Angles Arkussinus/1(z_I_Ground_m)
  Subsystem2/1(r_I_IK_m [3x1]) -> Bus Creator/1  "r_I_IK_m"
  Subsystem2/2(v_I_IK_mps [3x1]) -> Bus Creator/2  "v_I_IK_mps"
  Subsystem2/13(v_I_IAji_mps [3x4]) -> Bus Creator/13  "v_I_IAji_mps"
  Subsystem2/7(v_K_IK_mps [3x1]) -> Bus Creator/7  "v_K_IK_mps"
  Subsystem2/8(a_K_IK_mps2 [3x1]) -> Bus Creator/8  "a_K_IK_mps2"
  Bus Selector8/1 -> Bus Creator12/1  "<phi_IK_rad>"
  Bus Selector1/1 -> Rotation Angular Velocities VehicleFixed to TireFixed/1(omega_K_IK_radps)  "<omega_K_IK_radps>"
  Bus Selector6/1 -> Subsystem1/4(gamma-tau-nu_rad)  "<gamma-tau-nu_rad>"
  Bus Creator4/1 -> Bus Selector7/1
  Bus Creator5/1 -> SimDualTrackModel/1
  Bus Creator1/1 -> Bus Selector30/1, Bus Selector14/1, Bus Selector6/1, Bus Selector5/1, Bus Selector29/1
  Subsystem2/16(A_K_I [3x3]) -> Bus Creator/16  "A_K_I"
  Subsystem2/12(r_I_IAji_m [3x4]) -> Bus Creator/12  "r_I_IAji_m"
  Subsystem11/5(re_ji_m) -> Bus Creator2/3  "re_ji_m"
  Bus Selector7/1 -> Bus Creator10/3, Rotation Hardpoint Forces to VehicleFixed/1(F_F_Aji_N)  "<F_F_Aji_N>"
  Bus Selector7/2 -> Bus Creator10/4, Rotation Hardpoint Moments to VehicleFixed/1(T_F_Aji_Nm)  "<T_F_Aji_Nm>"
  Rotation Hardpoint Position from InertialFixed/1(r_F_IAji_m) -> Bus Creator6/1  "r_F_IAji_m"
  Rotation Hardpoint Forces to VehicleFixed/1(F_K_Aji_N) -> Bus Creator10/1, Subsystem3/4(F_K_Aji_N)  "F_K_Aji_N"
  Rotation Hardpoint Moments to VehicleFixed/1(T_K_Aji_Nm) -> Bus Creator10/2, Subsystem3/5(T_K_Aji_Nm)  "T_K_Aji_Nm"
  Bus Selector5/1 -> Rotation Velocities to TireFixed/1(v_F_IRji_mps)  "<v_F_IRji_mps>"
  Rotation Velocities to TireFixed/1(v_Tji_Rji_mps) -> Subsystem1/3(v_Tji_Rji_mps)  "v_Tji_Rji_mps"
  Bus Selector10/1 -> Selector21/1, Selector37/1, Selector3/1  "<phi_IK_rad>"
  Constant2/1 -> Computation Road Inclination Angles Arkussinus/2(l_WheelbaseFB_m)
  Constant5/1 -> Computation Road Inclination Angles Arkussinus/3(w_TrackFB_m)
  Bus Selector13/2 -> Rotation Hardpoint Velocities from VehicleFixed/1(v_K_IAji_mps)  "<v_K_IAji_mps>"
  Signal Specification2/1 -> Bus Creator12/2, Scope/1  "chi_IO_rad"
  Bus Selector13/1 -> Rotation Hardpoint Position from InertialFixed/1(r_I_IAji_m)  "<r_I_IAji_m>"
  Bus Selector4/1 -> Rotation Road Displacement InertialFrame to TireFixed/4(r_I_IAji_m)  "<r_I_IAji_m>"
  Bus Selector14/1 -> Rotation Road Displacement InertialFrame to TireFixed/5(h_ji_m)  "<h_ji_m>"
  Bus Selector15/1 -> Rotation Road Displacement InertialFrame to TireFixed/6(re_ji_m)  "<re_ji_m>"
  Bus Selector16/1 -> Subsystem/1(r_F_IAji_m)  "<r_F_IAji_m>"
  Bus Selector16/2 -> Subsystem/2(v_F_IAji_mps)  "<v_F_IAji_mps>"
  Bus Creator6/1 -> Bus Selector16/1
  Subsystem11/7(kappa_ji) -> Bus Creator2/5  "kappa_ji"
  Subsystem11/8(alpha_ji_rad) -> Bus Creator2/6  "alpha_ji_rad"
  Rotation Road Displacement InertialFrame to TireFixed/3(r_I_ITji_m) -> Bus Creator14/2  "r_I_ITji_m"
  Subsystem11/1(F_Tji_Tji_N) -> Rotation Forces from TireFixed/1(F_Tji_Tji_N), Bus Creator13/1  "F_Tji_Tji_N"
  Rotation Hardpoint Velocities from VehicleFixed/1(v_F_IAji_mps) -> Bus Creator6/2  "v_F_IAji_mps"
  Rotation Angular Velocities VehicleFixed to TireFixed/1(omega_Tji_ITji_radps) -> Subsystem1/5(omega_Tji_ITji_radps)  "omega_Tji_ITji_radps"
  Signal Specification5/1 -> Rotation RoadVerticalDisplacement InertialFrame to TireFixed/1(z_I_Ground_m), Rotation Road Displacement InertialFrame to TireFixed/1(z_I_Ground_m)
  Subsystem4/3(F_F_Rji_N) -> Bus Creator8/1  "F_F_Rji_N"
  delta_Wheel_rad [1x4]/1 -> Bus Creator12/3  "delta_ji_rad"
  Rotation Forces from TireFixed/1(F_F_Tji_N) -> Bus Creator13/3, Bus Creator3/1  "F_F_Tji_N"
  Rotation Moments from TireFixed/1(T_F_Tji_Nm) -> Bus Creator13/4, Bus Creator3/2  "T_F_Tji_Nm"
  Rotation Vertical Position TireFixed to RearAxleFixed z-down/1(rz_F_Rji_m) -> Bus Creator2/1  "rz_F_Rji_m"
  Rotation Vertical Velocity TireFixed to RearAxleFixed z-down/1(vz_F_Rji_mps) -> Bus Creator2/2  "vz_F_Rji_m"
  Subsystem/1(VehP [3x4]) -> Suspension System/1(VehP [3x4])
  Subsystem/2(VehV [3x4]) -> Suspension System/2(VehV [3x4])
  Subsystem/3(StrgAngF [1x2]) -> Suspension System/3(StrgAngF [1x2])
  Subsystem/4(WhlPz [1x4]) -> Suspension System/4(WhlPz [1x4])
  Subsystem/5(WhlRe [1x4]) -> Suspension System/5(WhlRe [1x4])
  Subsystem/6(WhlVz [1x4]) -> Suspension System/6(WhlVz [1x4])
  Subsystem/7(WhlFx [1x4]) -> Suspension System/7(WhlFx [1x4])
  Subsystem/8(WhlFy [1x4]) -> Suspension System/8(WhlFy [1x4])
  Subsystem/9(WhlM [3x4]) -> Suspension System/9(WhlM [3x4])
  Suspension System/1(VehF [3x4]) -> Subsystem4/1(VehF [3x4])
  Suspension System/2(VehM [3x4]) -> Subsystem4/2(VehM [3x4])
  Suspension System/3(WhlF [3x4]) -> Subsystem4/3(WhlF [3x4])
  Suspension System/4(WhlV [3x4]) -> Subsystem4/4(WhlV [3x4])
  Suspension System/5(WhlAng [3x4]) -> Subsystem4/5(WhlAng [3x4])
  Suspension System/6(SuspH [1x4]) -> Subsystem4/6(SuspH [1x4])
  Subsystem4/1(F_F_Aji_N) -> Bus Creator4/1  "F_F_Aji_N"
  Subsystem4/2(T_F_Aji_Nm) -> Bus Creator4/2  "T_F_Aji_Nm"
  Subsystem4/6(h_ji_m) -> Bus Creator1/3  "h_ji_m"
  Subsystem4/4(v_F_IRji_mps) -> Bus Creator1/1  "v_F_IRji_mps"
  Constant13/1 -> Vector Concatenate/1
  Constant14/1 -> Vector Concatenate/2
  Selector3/1 -> Vector Concatenate/3
  Selector37/1 -> Computation Road Inclination Angles Arkussinus/4(phiz_IK_rad)
  Vector Concatenate/1 -> Switch Off/On Road Inclination Angles/1
  Selector6/1 -> Computation Road Inclination Angles Arkustangens/2(rx_I_IAji_m)
  Selector20/1 -> Computation Road Inclination Angles Arkustangens/3(ry_I_IAji_m)
  Selector21/1 -> Computation Road Inclination Angles Arkustangens/4(phiz_IK_rad)
  Computation Road Inclination Angles Arkussinus/1(chi) -> Switch Computation Road Inclination Angles/1
  Computation Road Inclination Angles Arkustangens/1(chi) -> Switch Computation Road Inclination Angles/2
  Subsystem2/9(vdot_K_IK_mps2 [3x1]) -> Bus Creator/9  "vdot_K_IK_mps2"
  Subsystem3/5(MSusp [3x4]) -> Vehicle Body/5(MSusp [3x4])
  Combined Slip Wheels/1(Fx [1x4]) -> Subsystem11/1(Fx [1x4])
  Combined Slip Wheels/2(Fy [1x4]) -> Subsystem11/2(Fy [1x4])
  Combined Slip Wheels/3(Fz [1x4]) -> Subsystem11/3(Fz [1x4])
  Combined Slip Wheels/5(My [1x4]) -> Subsystem11/5(My [1x4])
  Combined Slip Wheels/6(Mz [1x4]) -> Subsystem11/6(Mz [1x4])
  Combined Slip Wheels/7(z [1x4]) -> Subsystem11/7(z [1x4])
  Combined Slip Wheels/8(zdot [1x4]) -> Subsystem11/8(zdot [1x4])
  Combined Slip Wheels/9(Re [1x4]) -> Subsystem11/9(Re [1x4])
  Combined Slip Wheels/10(omega [1x4]) -> Subsystem11/10(omega [1x4])
  Combined Slip Wheels/11(Kappa [1x4]) -> Subsystem11/11(Kappa [1x4])
  Subsystem11/2(T_Tji_Tji_Nm) -> Rotation Moments from TireFixed/1(T_Tji_Tji_Nm), Bus Creator13/2  "T_Tji_Tji_Nm"
  Subsystem11/3(rz_Tji_Rji_m) -> Rotation Vertical Position TireFixed to RearAxleFixed z-down/1(rz_Tji_Rji_m)  "rz_Tji_Rji_m"
  p_Brake_Pa [1x4]/1 -> Subsystem1/1(p_Brake_Pa)
  T_Wheel_Nm [1x4]/1 -> Subsystem1/2(T_Wheel_Nm)
  lambda_Tji_muex [1x4]/1 -> Subsystem1/7(lambda_Tji_muex [1x4])
  lambda_Tji_muey [1x4]/1 -> Subsystem1/8(lambda_Tji_muey [1x4])
  Switch Off/On Transformation Ground Displacement/1 -> Subsystem1/9(z_Tji_Ground_m [1x4])
  Rotation RoadVerticalDisplacement InertialFrame to TireFixed/1(z_Tji_Ground_m) -> Switch Off/On Transformation Ground Displacement/1  "z_Tji_Ground_m"
  Rotation Road Displacement InertialFrame to TireFixed/1(z_Tji_Ground_m) -> Switch Off/On Transformation Ground Displacement/2  "z_Tji_Ground_m"
  Bus Creator8/1 -> Bus Selector17/1
  Bus Selector17/1 -> Subsystem1/6(F_F_Rji_N [3x4])  "<F_F_Rji_N>"
  Switch Computation Road Inclination Angles/1 -> Switch Off/On Road Inclination Angles/2
  Switch Off/On Road Inclination Angles/1 -> Signal Specification2/1
  Subsystem1/1(BrkPrs [1x4]) -> Combined Slip Wheels/1(BrkPrs [1x4])
  Subsystem1/2(AxlTrq [1x4]) -> Combined Slip Wheels/2(AxlTrq [1x4])
  Subsystem1/3(Vx [1x4]) -> Combined Slip Wheels/3(Vx [1x4])
  Subsystem1/4(Vy [1x4]) -> Combined Slip Wheels/4(Vy [1x4])
  Subsystem1/5(Camber [1x4]) -> Combined Slip Wheels/5(Camber [1x4])
  Subsystem1/6(YawRate [1x4]) -> Combined Slip Wheels/6(YawRate [1x4])
  Subsystem1/7(Prs [1x4]) -> Combined Slip Wheels/7(Prs [1x4])
  Subsystem1/8(Gnd [1x4]) -> Combined Slip Wheels/8(Gnd [1x4])
  Subsystem1/9(Fext [1x4]) -> Combined Slip Wheels/9(Fext [1x4])
  Subsystem1/10(ScaleFctrs [27x4]) -> Combined Slip Wheels/10(ScaleFctrs [27x4])
  Combined Slip Wheels/12(Alpha [1x4]) -> Subsystem11/12(Alpha [1x4])
  Computation Transformation Matrices/1(A_K_I) -> Bus Creator9/1  "A_K_I"
  Computation Transformation Matrices/2(A_K_F) -> Bus Creator9/2  "A_K_F"
  Computation Transformation Matrices/3(A_F_I) -> Bus Creator9/3  "A_F_I"
  Computation Transformation Matrices/4(A_Rfl_F) -> Bus Creator9/4  "A_Rfl_F"
  Computation Transformation Matrices/5(A_Rfr_F) -> Bus Creator9/5  "A_Rfr_F"
  Computation Transformation Matrices/6(A_down_up) -> Bus Creator9/6  "A_down_up"
  Bus Selector/1 -> Rotation Hardpoint Forces to VehicleFixed/2(A_K_F)  "<A_K_F>"
  Bus Selector20/1 -> Rotation Hardpoint Moments to VehicleFixed/2(A_K_F)  "<A_K_F>"
  Bus Selector12/1 -> Rotation Hardpoint Velocities from VehicleFixed/2(A_K_F)  "<A_K_F>"
  Bus Selector21/1 -> Rotation Hardpoint Position from InertialFixed/2(A_K_I)  "<A_K_I>"
  Bus Selector21/2 -> Rotation Hardpoint Position from InertialFixed/3(A_F_I)  "<A_F_I>"
  Bus Selector24/1 -> Rotation Velocities to TireFixed/2(A_K_F)  "<A_K_F>"
  Bus Selector24/2 -> Rotation Velocities to TireFixed/3(A_Rfl_F)  "<A_Rfl_F>"
  Bus Selector24/3 -> Rotation Velocities to TireFixed/4(A_Rfr_F)  "<A_Rfr_F>"
  Bus Selector24/4 -> Rotation Velocities to TireFixed/5(A_down_up)  "<A_down_up>"
  Bus Selector25/1 -> Rotation Angular Velocities VehicleFixed to TireFixed/2(A_K_F)  "<A_K_F>"
  Bus Selector25/2 -> Rotation Angular Velocities VehicleFixed to TireFixed/3(A_down_up)  "<A_down_up>"
  Bus Selector26/1 -> Rotation Road Displacement InertialFrame to TireFixed/2(A_K_I)  "<A_K_I>"
  Bus Selector26/2 -> Rotation Road Displacement InertialFrame to TireFixed/3(A_F_I)  "<A_F_I>"
  Bus Selector27/1 -> Rotation Forces from TireFixed/2(A_K_F)  "<A_K_F>"
  Bus Selector27/2 -> Rotation Forces from TireFixed/3(A_Rfl_F)  "<A_Rfl_F>"
  Bus Selector27/3 -> Rotation Forces from TireFixed/4(A_Rfr_F)  "<A_Rfr_F>"
  Bus Selector27/4 -> Rotation Forces from TireFixed/5(A_down_up)  "<A_down_up>"
  Bus Selector28/1 -> Rotation Moments from TireFixed/2(A_K_F)  "<A_K_F>"
  Bus Selector28/2 -> Rotation Moments from TireFixed/3(A_Rfl_F)  "<A_Rfl_F>"
  Bus Selector28/3 -> Rotation Moments from TireFixed/4(A_Rfr_F)  "<A_Rfr_F>"
  Bus Selector28/4 -> Rotation Moments from TireFixed/5(A_down_up)  "<A_down_up>"
  Bus Selector22/1 -> Selector20/1, Selector6/1  "<r_I_IAji_m>"
  Subsystem2/17(F_K_g_N [3x1]) -> Bus Creator11/1  "F_K_g_N"
  Subsystem2/19(T_K_d_Nm [3x1]) -> Bus Creator11/3  "T_K_d_Nm"
  Subsystem2/20(F_K_sum_N [3x1]) -> Bus Creator11/4  "F_K_sum_N"
  Subsystem2/21(T_K_sum_Nm [3x1]) -> Bus Creator11/5  "T_K_sum_Nm"
  Subsystem3/4(FSusp [3x4]) -> Vehicle Body/4(FSusp [3x4])
  Vehicle Body/1(InertFrm.Cg.Disp [3x1]) -> Subsystem2/1(InertFrm.Cg.Disp [3x1])
  Vehicle Body/2(InertFrm.Cg.Vel [3x1]) -> Subsystem2/2(InertFrm.Cg.Vel [3x1])
  Vehicle Body/3(InertFrm.Cg.Ang [3x1]) -> Subsystem2/3(InertFrm.Cg.Ang [3x1])
  Vehicle Body/4(InertFrm.Axl.Disp [3x4]) -> Subsystem2/4(InertFrm.Axl.Disp [3x4])
  Vehicle Body/5(InertFrm.Axl.Vel [3x4]) -> Subsystem2/5(InertFrm.Axl.Vel [3x4])
  Vehicle Body/6(BdyFrm.Cg.Vel [3x1]) -> Subsystem2/6(BdyFrm.Cg.Vel [3x1])
  Vehicle Body/7(BdyFrm.Cg.AngVel [3x1]) -> Subsystem2/7(BdyFrm.Cg.AngVel [3x1])
  Vehicle Body/8(BdyFrm.Cg.Acc [3x1]) -> Subsystem2/8(BdyFrm.Cg.Acc [3x1])
  Vehicle Body/9(BdyFrm.Cg.AccRel [3x1]) -> Subsystem2/9(BdyFrm.Cg.AccRel [3x1])
  Vehicle Body/10(BdyFrm.Axl.Disp [3x4]) -> Subsystem2/10(BdyFrm.Axl.Disp [3x4])
  Vehicle Body/11(BdyFrm.Axl.Vel [3x4]) -> Subsystem2/11(BdyFrm.Axl.Vel [3x4])
  Vehicle Body/12(BdyFrm.Cg.DCM [3x3]) -> Subsystem2/12(BdyFrm.Cg.DCM [3x3])
  Vehicle Body/13(BdyFrm.Forces.Grvty [3x1]) -> Subsystem2/13(BdyFrm.Forces.Grvty [3x1])
  Vehicle Body/14(BdyFrm.Forces.Drag [3x1]) -> Subsystem2/14(BdyFrm.Forces.Drag [3x1])
  Vehicle Body/15(BdyFrm.Moments.Drag [3x1]) -> Subsystem2/15(BdyFrm.Moments.Drag [3x1])
  Vehicle Body/16(BdyFrm.Forces.Body [3x1]) -> Subsystem2/16(BdyFrm.Forces.Body [3x1])
  Vehicle Body/17(BdyFrm.Moments.Body [3x1]) -> Subsystem2/17(BdyFrm.Moments.Body [3x1])
  Subsystem2/11(alpha_K_IK_radps2 [3x1]) -> Bus Creator/11  "alpha_K_IK_radps2"
  Subsystem2/3(a_I_IK_mps2 [3x1]) -> Bus Creator/3  "a_I_IK_mps2"
  Subsystem2/5(omega_I_IK_radps [3x1]) -> Bus Creator/5  "omega_I_IK_radps"
  Subsystem2/6(alpha_I_IK_radps2 [3x1]) -> Bus Creator/6  "alpha_I_IK_radps2"
  Bus Creator11/1 -> Rearrange Force Bus/1(VehicleForces)  "VehicleForces"
  Bus Creator10/1 -> Rearrange Force Bus/2(SuspensionForces)  "SuspensionForces"
  Bus Creator13/1 -> Rearrange Force Bus/3(TireForces)  "TireForces"
  Rearrange Force Bus/1(Force) -> Bus Creator5/6  "SimForce"
  Rotation Road Displacement InertialFrame to TireFixed/2(r_I_IRji_m) -> Bus Creator14/1  "r_I_IRji_m"
  Subsystem3/1(FExt [3x1]) -> Vehicle Body/1(FExt [3x1])
  Subsystem3/2(MExt [3x1]) -> Vehicle Body/2(MExt [3x1])
  Subsystem3/3(WindXYZ [3x1]) -> Vehicle Body/3(WindXYZ [3x1])
  Bus Creator12/1 -> Bus Selector23/1, Computation Chassis Coordinate System/1(TransformationAngles), Bus Selector19/1  "TransformationAngles"
  Bus Selector19/1 -> Computation Transformation Matrices/1(phi)  "<phi_IK_rad>"
  Bus Selector19/2 -> Computation Transformation Matrices/2(chi)  "<chi_IO_rad>"
  Bus Selector19/3 -> Computation Transformation Matrices/3(delta)  "<delta_ji_rad>"
  Bus Selector23/1 -> Subsystem/3(delta_ji_rad)  "<delta_ji_rad>"
  Computation Chassis Coordinate System/1(Chassis) -> Bus Creator5/2  "SimChassis"
  Bus Selector29/1 -> Bus Creator5/3  "SimSuspension"
  Bus Selector30/1 -> Bus Creator14/3  "<v_F_IRji_mps>"
  Bus Creator14/1 -> Bus Selector31/1
  Bus Selector31/2 -> Bus Creator2/8  "<r_I_ITji_m>"
  Bus Selector31/3 -> Bus Creator2/9  "<v_F_IRji_mps>"
  Bus Selector31/1 -> Bus Creator2/7  "<r_I_IRji_m>"
  Combined Slip Wheels/4(Mx [1x4]) -> Subsystem11/4(Mx [1x4])
  Subsystem2/18(F_K_d_N [3x1]) -> Bus Creator11/2  "F_K_d_N"
  Switch Off/On Correction Horizontal Dynamics Wheel Inertia according d'Alembert/1 -> Add/1
  Constant6/1 -> Wheel Inertia according d'Alembert/3(m_WheelsFB_kg)
  Bus Selector32/1 -> Memory/1  "<a_K_IK_mps2>"
  Signal Specification4/1 -> Switch Off/On Correction Horizontal Dynamics Wheel Inertia according d'Alembert/2
  Bus Selector33/1 -> Memory1/1  "<A_K_F>"
  Constant15/1 -> Switch Off/On Correction Horizontal Dynamics Wheel Inertia according d'Alembert/1
  Memory/1 -> Wheel Inertia according d'Alembert/1(a_K_IK_mps2)
  Bus Creator9/1 -> Bus Selector28/1, Bus Selector27/1, Bus Selector24/1, Bus Selector26/1, Bus Selector25/1, Bus Selector20/1, Bus Selector/1, Bus Selector33/1, Bus Selector21/1, Bus Selector12/1, Computation Chassis Coordinate System/2(Transformation), Bus Creator5/5
  Wheel Inertia according d'Alembert/1(F_K_dAlembert_N) -> Signal Specification4/1
  Bus Creator/1 -> Bus Selector32/1, Bus Selector13/1, Bus Creator5/1, Bus Selector8/1, Bus Selector4/1, Bus Selector1/1, Bus Selector10/1, Bus Selector22/1
  Memory1/1 -> Wheel Inertia according d'Alembert/2(A_K_F)
  F_K_Extern_N [3x1]/1 -> Add/2
